simulink model "Kalman_model"  (R2017a)
settings: Solver=VariableStepAuto  StartTime=0.0  StopTime=1000  RelTol=1e-3
values from neighbouring files (symbols this model uses):
  P_0 = eye(6)*100    [Kalman_setup.m]
  Ts = 0.05    [Kalman_setup.m]
  x_0 = zeros(6,1)    [Kalman_setup.m]
settings Model: Creator=sverreknutsen  LastModifiedBy=sverreknutsen

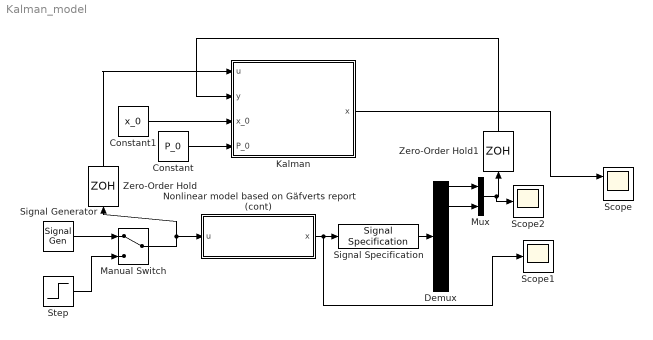
== system Kalman_model ==
  Constant : Constant  Value=P_0
  Constant1 : Constant  Value=x_0
  Demux : Demux  Outputs=6
  Kalman : MATLAB Function  TreatAsAtomicUnit=on
  Manual Switch : ManualSwitch
  Mux : Mux  Inputs=2
  Nonlinear model based on Gäfverts report (cont) : Subsystem
  Scope : Scope  NumInputPorts=2
  Scope1 : Scope
  Scope2 : Scope
  Signal Generator : SignalGenerator  WaveForm=square  Amplitude=[1,1]'  Units=rad/sec
  Signal Specification : SignalSpecification  Dimensions=[6,1]
  Step : Step  Before=[0 0]'  After=[1,1]'  SampleTime=0
  Zero-Order Hold : ZeroOrderHold  SampleTime=Ts
  Zero-Order Hold1 : ZeroOrderHold  SampleTime=Ts
  wires:
  Nonlinear model based on Gäfverts report (cont)/1(x) -> Scope1/1, Signal Specification/1
  Signal Specification/1 -> Demux/1
  Constant/1 -> Kalman/4(P_0)
  Constant1/1 -> Kalman/3(x_0)
  Mux/1 -> Scope2/1, Zero-Order Hold1/1
  Demux/1 -> Mux/1
  Demux/2 -> Mux/2
  Kalman/1(x) -> Scope/1
  Zero-Order Hold1/1 -> Kalman/2(y)
  Zero-Order Hold/1 -> Kalman/1(u)
  Step/1 -> Manual Switch/2
  Manual Switch/1 -> Zero-Order Hold/1, Nonlinear model based on Gäfverts report (cont)/1(u)
  Signal Generator/1 -> Manual Switch/1

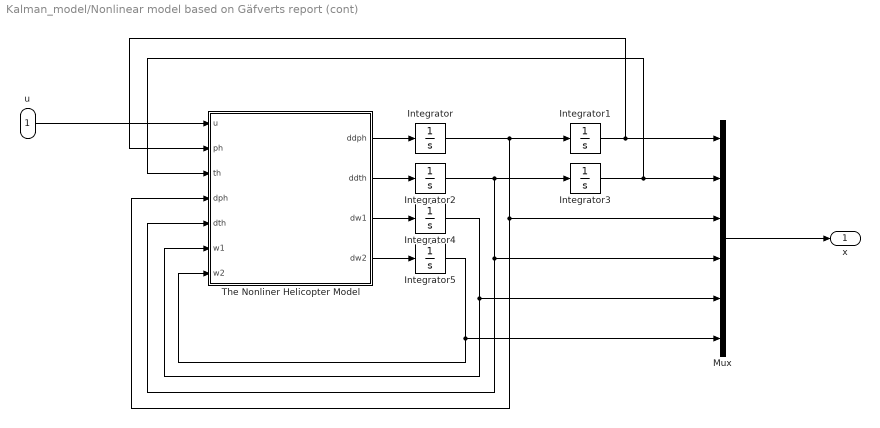
== system Kalman_model/Nonlinear model based on Gäfverts report (cont) ==
  u : Inport
  Integrator{,1..5} (6 alike) : Integrator
  Mux : Mux  Inputs=6
  The Nonliner Helicopter Model : MATLAB Function  TreatAsAtomicUnit=on
  x : Outport
  wires:
  u/1 -> The Nonliner Helicopter Model/1(u)
  The Nonliner Helicopter Model/1(ddph) -> Integrator/1
  Integrator/1 -> Mux/3, The Nonliner Helicopter Model/4(dph), Integrator1/1
  The Nonliner Helicopter Model/2(ddth) -> Integrator2/1
  Integrator2/1 -> Integrator3/1, The Nonliner Helicopter Model/5(dth), Mux/4
  The Nonliner Helicopter Model/3(dw1) -> Integrator4/1
  The Nonliner Helicopter Model/4(dw2) -> Integrator5/1
  Integrator5/1 -> The Nonliner Helicopter Model/7(w2), Mux/6
  Integrator4/1 -> The Nonliner Helicopter Model/6(w1), Mux/5
  Integrator1/1 -> The Nonliner Helicopter Model/2(ph), Mux/1
  Integrator3/1 -> Mux/2, The Nonliner Helicopter Model/3(th)
  Mux/1 -> x/1

== matlab function Kalman_model/Nonlinear model based on Gäfverts report (cont)/The Nonliner Helicopter Model ==
  data: u input; ddph output; ph input; th input; dph input; dth input; w1 input; w2 input; ddth output; dw1 output; dw2 output
function [ddph, ddth, dw1, dw2] = fcn(u, ph, th, dph, dth, w1, w2)
% Implementation of the non-linear integration model derived in the
% technical report "Modelling of the ETH Helicopter Laboratory Process"
% by Magnus Gäfvert, implemented by Marcus Greiff for the project course in
% FRTN01/FRTN15 2018-03-18. The notation and nomenclature vollows the
% report, however, the state vector is defined as
%
%   $x \triangleq [phi; theta; \dot{phi}; \dot{theta}; \omega_1; \omega_2]$
%
% The parameters in Gäfverts report are hard coded in the non-linear model,
% but will be made more general in future revisions.

%% Parameters
% Weights
ml = 0.280;  % [kg]
m1 = 0.3792; % [kg]
m2 = 0.1739; % [kg]
mw = 0.158;  % [kg]
m  = ml + m1 + m2 + mw; % [kg] (eq. 24)

% Distances
l1 = 0.1995; % [m]
l2 = 0.1743; % [m]
lw = 0.090;  % [m]
h  = 0.0298; % [m]
lc = (m1*(l1-l2)+m1*l1-m2*l2-mw*lw)/m; % [m] (eq. 27)

% Inertial parameters
g = 9.81; % [m/s^2]
Ja = 0;   % [] (eq. 26)
Jl = (ml/3)*((l1^3+l2^3)/(l1+l2))+m1*l1^2+m2*l2^2+mw*lw^2; % [] (eq. 25)

% Time, motor and aerodynamics constants
k1 = 1.00e-2; % [Vs/rad]
k2 = 1.39e-2; % [Vs/rad]
C1 = 2.50e-5; % [Ns^/rad^2]
C2 = 1.58e-6; % [Ns^/rad^2]
D1 = 2.90e-7; % [Nms^/rad^2]
D2 = 1.76e-7; % [Nms^/rad^2]
T1 = 1.10;    % [s]
T2 = 0.33;    % [s]

%% Pre-computation of angles and extraction of states
cth = cos(th);
sth = sin(th);
u1 = u(1);
u2 = u(2);

%% Integration model
ddph = (cth^2*Jl - 2*h*cth*sth*m*lc + h^2*sth^2*m + Ja)\...
       (2*cth*sth*dph*dth*Jl - 2*h*(sth^2-cth^2)*dph*dth*m*lc - ...
	2*h^2*sth*cth*dph*dth*m + D1*w1*abs(w1)*cth + l2*cth*C2*w2*abs(w2));
ddth = (Jl + h^2*m)\...
       (-cth*sth*dph^2*Jl - h*(-sth^2+cth^2)*dph^2*m*lc - g*cth*m*lc ...
	+ h^2*sth*cth*dph^2*m + m*g*h*sth + l1*C1*w1*abs(w1) + D2*w2*abs(w2));
dw1 = -w1/T1 + u1/(k1*T1);
dw2 = -w2/T2 + u2/(k2*T2);

== matlab function Kalman_model/Kalman ==
  data: u input; x output; y input; x_0 input; P_0 input
function x = regular_kalman(u,y,x_0,P_0)
persistent x_hat;
persistent P;
if(isempty(x_hat))
    x_hat=x_0;
    P=P_0;
end
coder.extrinsic('updateKalman');
[x_hat,P]=updateKalman(x_hat,u,y,P);
x=x_hat;
